simulink model "exp7Fw"  (R2024a)
settings: Solver=VariableStepAuto  StartTime=0.0  StopTime=0.05  RelTol=1e-3
libraries: spsDetailedThyristorLib x6, spsVoltageMeasurementLib x4, spsACVoltageSourceLib x3, spsCurrentMeasurementLib x1, spsSeriesRLCBranchLib x1, sps_lib x1
settings Model: Creator=おもい  LastModifiedBy=おもい

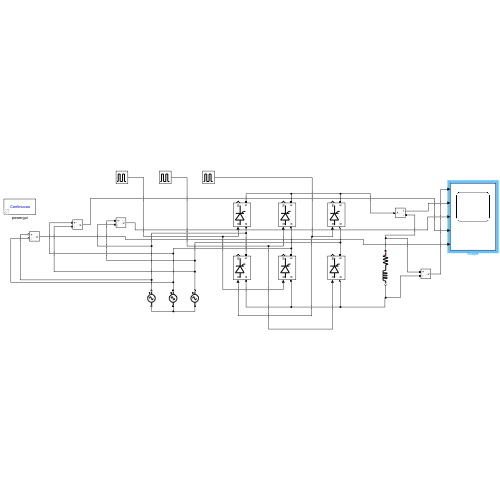
[thumbnail: Simulink's stored preview of the top-level diagram]
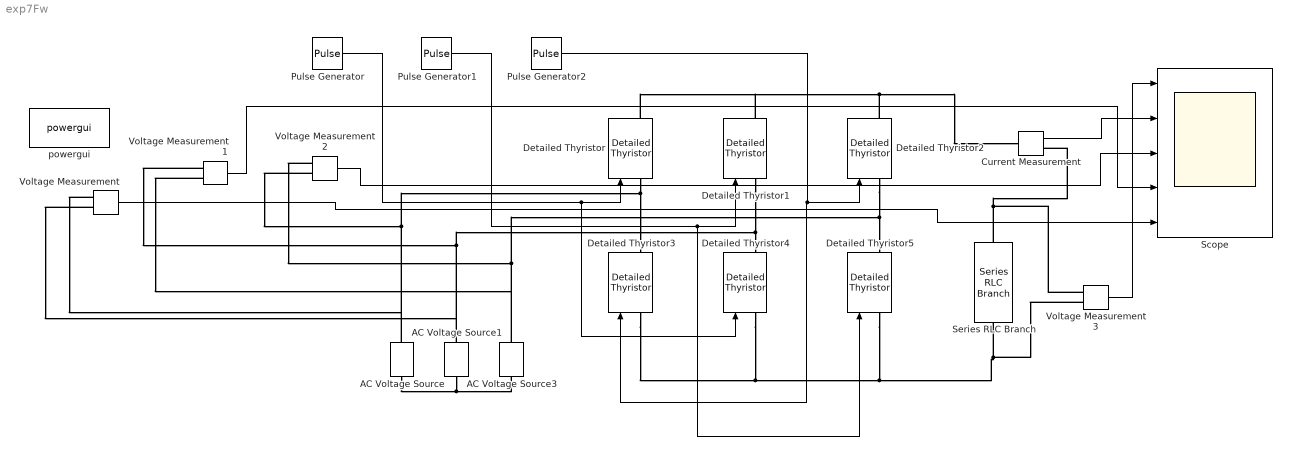
== system exp7Fw ==
  AC Voltage Source : spsACVoltageSourceLib/AC Voltage Source  Amplitude=230  Phase=0  Frequency=50  SampleTime=0  Measurements=None  BusType=swing  Pref=10e3  Qref=0  Qmin=-inf  Qmax=+inf
  AC Voltage Source1 : spsACVoltageSourceLib/AC Voltage Source  Amplitude=230  Phase=-120  Frequency=50  SampleTime=0  Measurements=None  BusType=swing  Pref=10e3  Qref=0  Qmin=-inf  Qmax=+inf
  AC Voltage Source3 : spsACVoltageSourceLib/AC Voltage Source  Amplitude=230  Phase=120  Frequency=50  SampleTime=0  Measurements=None  BusType=swing  Pref=10e3  Qref=0  Qmin=-inf  Qmax=+inf
  Current Measurement : spsCurrentMeasurementLib/Current Measurement  PhasorSimulation=off  OutputType=Complex  PSBequivalent=0
  Detailed Thyristor{,1..5} (6 alike) : spsDetailedThyristorLib/Detailed Thyristor  Ron=0.001  Lon=1e-3  Vf=0.8  IL=0.1  Tq=100e-6  IC=0  Rs=inf  Cs=inf  Measurements=on
      settings: LibrarySourceBlock=sps_lib/Power Electronics/Detailed Thyristor
  Pulse Generator : DiscretePulseGenerator  PulseType=Time based  Amplitude=10  Period=0.02  PulseWidth=5  PhaseDelay=((.02*90)/360)
  Pulse Generator1 : DiscretePulseGenerator  PulseType=Time based  Amplitude=10  Period=0.02  PulseWidth=5  PhaseDelay=(.02*210)/360
  Pulse Generator2 : DiscretePulseGenerator  PulseType=Time based  Amplitude=10  Period=0.02  PulseWidth=5  PhaseDelay=(.02*330)/360
  Scope : Scope  NumInputPorts=5
  Series RLC Branch : spsSeriesRLCBranchLib/Series RLC Branch  LConnTagsString=__new0  RConnTagsString=__new0  BranchType=RL  Resistance=50  Inductance=.0001  SetiL0=off  InitialCurrent=0  Capacitance=1e-6  Setx0=off  InitialVoltage=0  Measurements=None
  Voltage Measurement{,1..3} (4 alike) : spsVoltageMeasurementLib/Voltage Measurement  PhasorSimulation=off  OutputType=Complex  PSBequivalent=0
  powergui : sps_lib/powergui  Priority=1  SimulationMode=Continuous  SampleTime=50e-6  frequency=60  Iterations=50  frequencyindice=50  Pbase=100e6  ErrMax=1e-4  UnitsV=kV  UnitsW=MW  buscounter=0  FunctionMessages=off  echomessages=off  EnableUseOfTLC=off  CurrentSourceSwitches=off  DisableSnubberDevices=off  DisableRonSwitches=off  DisableVfSwitches=off  DisplayEquations=off  AutomaticDiscreteSolvers=off  SolverType=Tustin/Backward Euler (TBE)  Interpol=off  ExternalGateDelay=off  methode=off  Ts=100  x0status=blocks  SPID=on  SwTol=0  HookPort=off  NonlinearTolerance=1e-4  nMaxIteration=100  ContinueOnMaxIteration=off  RestoreLinks=warning  ResistiveCurrentMeasurement=off  Frange=[0:2:500]  Ylog=off  Xlog=on  ShowGrid=off  save=off  variable=ZData  structure=0  ZoomFFT=off  StartTime=0.0  cycles=1  DisplayStyle=1  fundamental=60  FreqAxis=off  MaxFrequency=1000  frequencyindicesteady=1  RmsSteady=1  display=off
  wires:
  Pulse Generator/1 -> Detailed Thyristor4/1, Detailed Thyristor/1
  Pulse Generator2/1 -> Detailed Thyristor3/1, Detailed Thyristor2/1
  Pulse Generator1/1 -> Detailed Thyristor5/1, Detailed Thyristor1/1
  Current Measurement/1 -> Scope/2
  Voltage Measurement3/1 -> Scope/1
  Voltage Measurement2/1 -> Scope/3
  Voltage Measurement1/1 -> Scope/4
  Voltage Measurement/1 -> Scope/5
  connections:
  Detailed Thyristor2/RConn1 -- Detailed Thyristor/RConn1 -- Detailed Thyristor1/RConn1 -- Current Measurement/LConn1
  Detailed Thyristor/LConn1 -- Voltage Measurement/LConn1 -- AC Voltage Source/RConn1 -- Voltage Measurement2/LConn2 -- Detailed Thyristor3/RConn1
  Detailed Thyristor1/LConn1 -- Voltage Measurement/LConn2 -- AC Voltage Source1/RConn1 -- Voltage Measurement1/LConn1 -- Detailed Thyristor4/RConn1
  Detailed Thyristor2/LConn1 -- Voltage Measurement1/LConn2 -- AC Voltage Source3/RConn1 -- Voltage Measurement2/LConn1 -- Detailed Thyristor5/RConn1
  Detailed Thyristor3/LConn1 -- Detailed Thyristor4/LConn1 -- Detailed Thyristor5/LConn1 -- Voltage Measurement3/LConn2 -- Series RLC Branch/RConn1
  Series RLC Branch/LConn1 -- Voltage Measurement3/LConn1 -- Current Measurement/RConn1
  AC Voltage Source/LConn1 -- AC Voltage Source1/LConn1 -- AC Voltage Source3/LConn1
